simulink model "NewSync_Axial_Flux_Generator_Modelled"  (R2018a)
settings: Solver=ode1  StartTime=0.0  StopTime=1  FixedStep=1e-6  MaxStep=1e-6  RelTol=1e-3
PreLoadFcn:
  | Ts=1/1000
InitFcn:
  | Pref=2000;
  | D=4;
  | P=10;
  | Rd=5;
  | Rq=5;
  | Ld=2.094;
  | Lq= 0.8187;
  | Phi= 1.6
  | Pref = 2000;
  | J=4;
  | K=0.16;
  | c1= 0.5176;
  | c2= 116;
  | c3= 0.4;
  | c4= 5;
  | c5= 21;
  | c6= 0.0068;
  | Den= 1.225;
  | A= 2
  | Ts=1/1000
undefined symbols (not defined in the file): D1, Delta
libraries: powerlib x84, powerlib_meascontrol x17, simulink x13, re_lib x1, electricdrivelib x1, pePowerMeasurement x1
(part 2 of 2)

== system NewSync_Axial_Flux_Generator_Modelled/Utility Grid ==
  120 kV / 25 kV 47 MVA : powerlib/Elements/Three-Phase Transformer (Two Windings)  Winding1Connection=Yg  Winding2Connection=Delta (D1)  CoreType=Three single-phase transformers  SetSaturation=off  Hysteresis=off  DataFile='basic_model'  SetInitialFlux=off  Measurements=None  UNITS=pu  NominalPower=[47e6 60 ]  Winding1="[ 120e3  0.08/30   0.08 ]"  Winding2="[ 25e3  0.08/30  0.08]"  Rm=500  Lm=500  L0=0.5  Saturation="[ 0,0  ;  0.005,1.2  ;  1.0,1.4 ]"  InitialFluxes=[ 0.8 , -0.8 , 0.7 ]  MoreParameters=off  BreakLoop=off  DataType=off  TransfoNumber=0
  120kV 2500MVA : powerlib/Electrical Sources/Three-Phase Source  InternalConnection=Yg  VoltagePhases=off  Voltage=120e3  PhaseAngle=0  Voltage_phases=[25e3 25e3 25e3]/sqrt(3)  PhaseAngles_phases=[0 -120 +120]  Frequency=60  NonIdealSource=on  SpecifyImpedance=on  Resistance=0.8929  Inductance=16.58e-3  ShortCircuitLevel=2500e6  BaseVoltage=120e3  XRratio=7  BusType=swing  Pref=0  Qref=0  Prefabc=[10e3, 10e3, 10e3]  Qrefabc=[0, 0, 0]  Qmin=-inf  Qmax=inf
  14-km Feeder : powerlib/Elements/Distributed Parameters Line  Phases=3  Frequency=60  Resistance=[0.1153 0.413]  Inductance=[1.05e-3 3.32e-3]  Capacitance=[11.33e-009 5.01e-009]  Length=14  x1=[-5.8e-05 -8.35000296312306e-11 0 0;-5.7e-05 -8.31426687600871e-11 0 0;-5.6e-05 -8.27852960725161e-11 0 0;-5.5e-05 -8.24279116193083e-11 0 0;-5.4e-05 -8.2070515451256e-11 0 0;-5.3e-05 -8.1713107619153e-11 0 0;-5.2e-05 -8.13556881737952e-11 0 0;-5.1e-05 -8.09982571659797e-11 0 0;-5e-05 -8.06408146465055e-11 0 0;-4.9e-05 -8.02833606661731e-11 -3803.81447652567 -24026.5579932896;-4.8e-05 -7.99258952757846e-11 -3794.75640746685 -24027.9902901746;-4.7e-05 -7.9568418526144e-11 -3785.69779908852 -24029.4191721463;-4.6e-05 -7.92109304680566e-11 -3776.63865267811 -24030.8446390016;-4.5e-05 -7.88534311523294e-11 -3767.57896952312 -24032.266690538;-4.4e-05 -7.84959206297711e-11 -3758.51875091113 -24033.6853265533;-4.3e-05 -7.81383989511919e-11 -3749.45799812981 -24035.100546846;-4.2e-05 -7.77808661674036e-11 -3740.39671246689 -24036.5123512148;-4.1e-05 -7.74233223292195e-11 -3731.33489521017 -24037.9207394592;-4e-05 -7.70657674874547e-11 -3722.27254764756 -24039.3257113789;-3.9e-05 -7.67082016929256e-11 -3713.209671067 -24040.7272667744;-3.8e-05 -7.63506249964504e-11 -3704.14626675653 -24042.1254054463;-3.7e-05 -7.59930374488485e-11 -3695.08233600428 -24043.5201271961;-3.6e-05 -7.56354391009413e-11 -3686.01788009841 -24044.9114318254;-3.5e-05 -7.52778300035514e-11 -3676.9529003272 -24046.2993191366;-3.4e-05 -7.4920210207503e-11 -3667.88739797898 -24047.6837889324;-3.3e-05 -7.45625797636219e-11 -3658.82137434217 -24049.064841016;-3.2e-05 -7.42049387227354e-11 -3649.75483070523 -24050.4424751912;-3.1e-05 -7.38472871356721e-11 -3640.68776835674 -24051.8166912621;-3e-05 -7.34896250532625e-11 -3631.62018858533 -24053.1874890334;-2.9e-05 -7.31319525263381e-11 -3622.55209267969 -24054.5548683104;-2.8e-05 -7.27742696057324e-11 -3613.48348192861 -24055.9188288987;-2.7e-05 -7.241657634228e-11 -3604.41435762095 -24057.2793706045;-2.6e-05 -7.2058872786817e-11 -3595.34472104562 -24058.6364932343;-2.5e-05 -7.17011589901812e-11 -3586.27457349162 -24059.9901965953;-2.4e-05 -7.13434350032116e-11 -3577.20391624802 -24061.3404804952;-2.3e-05 -7.09857008767488e-11 -3568.13275060397 -24062.6873447419;-2.2e-05 -7.06279566616349e-11 -3559.06107784868 -24064.0307891442;-2.1e-05 -7.02702024087132e-11 -3549.98889927144 -24065.370813511;-2e-05 -6.99124381688286e-11 -3540.91621616161 -24066.7074176519;-1.9e-05 -6.95546639928273e-11 -3531.84302980861 -24068.0406013769;-1.8e-05 -6.91968799315571e-11 -3522.76934150195 -24069.3703644966;-1.7e-05 -6.8839086035867e-11 -3513.69515253121 -24070.6967068221;-1.6e-05 -6.84812823566077e-11 -3504.62046418602 -24072.0196281647;-1.5e-05 -6.81234689446308e-11 -3495.5452777561 -24073.3391283364;-1.4e-05 -6.77656458507897e-11 -3486.46959453125 -24074.6552071498;-1.3e-05 -6.74078131259391e-11 -3477.39341580131 -24075.9678644178;-1.2e-05 -6.70499708209349e-11 -3468.31674285622 -24077.2770999538;-1.1e-05 -6.66921189866345e-11 -3459.23957698596 -24078.5829135718;-1e-05 -6.63342576738967e-11 -3450.16191948062 -24079.8853050861;-9e-06 -6.59763869335815e-11 -3441.08377163032 -24081.1842743117;-8e-06 -6.56185068165503e-11 -3432.00513472528 -24082.479821064;-7e-06 -6.52606173736659e-11 -3422.92601005577 -24083.7719451588;-6e-06 -6.49027186557924e-11 -3413.84639891213 -24085.0606464126;-5e-06 -6.4544810713795e-11 -3404.76630258479 -24086.345924642;-4e-06 -6.41868935985407e-11 -3395.68572236422 -24087.6277796646;-3e-06 -6.38289673608972e-11 -3386.60465954098 -24088.906211298;-2e-06 -6.3471032051734e-11 -3377.5231154057 -24090.1812193606;-1e-06 -6.31130877219217e-11 -3368.44109124905 -24091.4528036713]  x2=[-5.8e-05 -3.28293887343002e-10 0 0;-5.7e-05 -3.27276455725141e-10 0 0;-5.6e-05 -3.26258977593998e-10 0 0;-5.5e-05 -3.25241453094177e-10 0 0;-5.4e-05 -3.24223882370293e-10 0 0;-5.3e-05 -3.23206265566964e-10 0 0;-5.2e-05 -3.22188602828817e-10 0 0;-5.1e-05 -3.21170894300484e-10 0 0;-5e-05 -3.20153140126605e-10 0 0;-4.9e-05 -3.19135340451824e-10 -3384.04949800626 -24234.37909601;-4.8e-05 -3.18117495420794e-10 -3374.91311206833 -24235.653130462;-4.7e-05 -3.17099605178173e-10 -3365.77624647999 -24236.9237204872;-4.6e-05 -3.16081669868627e-10 -3356.63890253978 -24238.190865905;-4.5e-05 -3.15063689636826e-10 -3347.50108154632 -24239.4545665353;-4.4e-05 -3.14045664627449e-10 -3338.36278479831 -24240.7148221985;-4.3e-05 -3.13027594985179e-10 -3329.22401359449 -24241.9716327156;-4.2e-05 -3.12009480854706e-10 -3320.08476923369 -24243.2249979079;-4.1e-05 -3.10991322380728e-10 -3310.9450530148 -24244.4749175972;-4e-05 -3.09973119707947e-10 -3301.80486623678 -24245.7213916059;-3.9e-05 -3.08954872981073e-10 -3292.66421019866 -24246.9644197569;-3.8e-05 -3.07936582344822e-10 -3283.52308619951 -24248.2040018736;-3.7e-05 -3.06918247943915e-10 -3274.38149553851 -24249.4401377796;-3.6e-05 -3.05899869923079e-10 -3265.23943951487 -24250.6728272994;-3.5e-05 -3.0488144842705e-10 -3256.09691942789 -24251.9020702578;-3.4e-05 -3.03862983600568e-10 -3246.95393657692 -24253.12786648;-3.3e-05 -3.0284447558838e-10 -3237.81049226139 -24254.3502157919;-3.2e-05 -3.01825924535237e-10 -3228.66658778077 -24255.5691180197;-3.1e-05 -3.00807330585899e-10 -3219.52222443463 -24256.7845729902;-3e-05 -2.99788693885132e-10 -3210.37740352258 -24257.9965805306;-2.9e-05 -2.98770014577705e-10 -3201.2321263443 -24259.2051404687;-2.8e-05 -2.97751292808395e-10 -3192.08639419954 -24260.4102526328;-2.7e-05 -2.96732528721987e-10 -3182.94020838812 -24261.6119168515;-2.6e-05 -2.95713722463269e-10 -3173.79357020991 -24262.810132954;-2.5e-05 -2.94694874177036e-10 -3164.64648096485 -24264.0049007702;-2.4e-05 -2.93675984008089e-10 -3155.49894195295 -24265.1962201301;-2.3e-05 -2.92657052101235e-10 -3146.35095447428 -24266.3840908645;-2.2e-05 -2.91638078601287e-10 -3137.20251982897 -24267.5685128045;-2.1e-05 -2.90619063653065e-10 -3128.05363931721 -24268.7494857818;-2e-05 -2.89600007401392e-10 -3118.90431423928 -24269.9270096286;-1.9e-05 -2.885809099911e-10 -3109.75454589548 -24271.1010841776;-1.8e-05 -2.87561771567024e-10 -3100.60433558621 -24272.2717092617;-1.7e-05 -2.86542592274007e-10 -3091.45368461191 -24273.4388847147;-1.6e-05 -2.85523372256898e-10 -3082.3025942731 -24274.6026103708;-1.5e-05 -2.8450411166055e-10 -3073.15106587035 -24275.7628860644;-1.4e-05 -2.83484810629823e-10 -3063.9991007043 -24276.9197116308;-1.3e-05 -2.82465469309582e-10 -3054.84670007565 -24278.0730869054;-1.2e-05 -2.81446087844698e-10 -3045.69386528515 -24279.2230117244;-1.1e-05 -2.80426666380049e-10 -3036.54059763362 -24280.3694859243;-1e-05 -2.79407205060516e-10 -3027.38689842196 -24281.5125093423;-9e-06 -2.78387704030988e-10 -3018.2327689511 -24282.6520818158;-8e-06 -2.77368163436359e-10 -3009.07821052206 -24283.7882031829;-7e-06 -2.76348583421528e-10 -2999.9232244359 -24284.9208732821;-6e-06 -2.753289641314e-10 -2990.76781199374 -24286.0500919525;-5e-06 -2.74309305710887e-10 -2981.61197449677 -24287.1758590335;-4e-06 -2.73289608304903e-10 -2972.45571324625 -24288.2981743652;-3e-06 -2.72269872058371e-10 -2963.29902954348 -24289.4170377881;-2e-06 -2.71250097116218e-10 -2954.14192468984 -24290.5324491431;-1e-06 -2.70230283623378e-10 -2944.98439998674 -24291.6444082717]  x3=[-5.8e-05 -9.39139589328699e-11 0 0;-5.7e-05 -9.39069853666868e-11 0 0;-5.6e-05 -9.38999984542268e-11 0 0;-5.5e-05 -9.38929981964829e-11 0 0;-5.4e-05 -9.38859845944499e-11 0 0;-5.3e-05 -9.38789576491248e-11 0 0;-5.2e-05 -9.38719173615061e-11 0 0;-5.1e-05 -9.38648637325944e-11 0 0;-5e-05 -9.38577967633923e-11 0 0;-4.9e-05 -9.3850716454904e-11 -27.3571063473752 -158.181189142487;-4.8e-05 -9.38436228081359e-11 -27.2974715013507 -158.191491287824;-4.7e-05 -9.38365158240962e-11 -27.2378327757468 -158.201770950623;-4.6e-05 -9.38293955037948e-11 -27.1781901790394 -158.212028129421;-4.5e-05 -9.38222618482438e-11 -27.118543719705 -158.222262822762;-4.4e-05 -9.3815114858457e-11 -27.0588934062207 -158.232475029191;-4.3e-05 -9.38079545354501e-11 -26.9992392470643 -158.242664747256;-4.2e-05 -9.38007808802408e-11 -26.9395812507138 -158.25283197551;-4.1e-05 -9.37935938938486e-11 -26.8799194256481 -158.262976712507;-4e-05 -9.3786393577295e-11 -26.8202537803463 -158.273098956805;-3.9e-05 -9.37791799316032e-11 -26.7605843232883 -158.283198706966;-3.8e-05 -9.37719529577985e-11 -26.7009110629545 -158.293275961555;-3.7e-05 -9.37647126569081e-11 -26.6412340078257 -158.303330719139;-3.6e-05 -9.37574590299609e-11 -26.5815531663834 -158.313362978289;-3.5e-05 -9.37501920779878e-11 -26.5218685471097 -158.32337273758;-3.4e-05 -9.37429118020216e-11 -26.4621801584869 -158.333359995588;-3.3e-05 -9.3735618203097e-11 -26.4024880089982 -158.343324750895;-3.2e-05 -9.37283112822506e-11 -26.3427921071271 -158.353267002085;-3.1e-05 -9.37209910405209e-11 -26.2830924613577 -158.363186747743;-3e-05 -9.37136574789482e-11 -26.2233890801748 -158.373083986461;-2.9e-05 -9.37063105985748e-11 -26.1636819720634 -158.382958716832;-2.8e-05 -9.36989504004449e-11 -26.1039711455094 -158.392810937451;-2.7e-05 -9.36915768856045e-11 -26.0442566089988 -158.402640646921;-2.6e-05 -9.36841900551015e-11 -25.9845383710186 -158.412447843842;-2.5e-05 -9.36767899099858e-11 -25.924816440056 -158.422232526821;-2.4e-05 -9.36693764513091e-11 -25.8650908245988 -158.431994694469;-2.3e-05 -9.3661949680125e-11 -25.8053615331354 -158.441734345396;-2.2e-05 -9.36545095974891e-11 -25.7456285741546 -158.451451478219;-2.1e-05 -9.36470562044587e-11 -25.6858919561457 -158.461146091558;-2e-05 -9.36395895020931e-11 -25.6261516875989 -158.470818184034;-1.9e-05 -9.36321094914535e-11 -25.5664077770043 -158.480467754272;-1.8e-05 -9.3624616173603e-11 -25.506660232853 -158.490094800901;-1.7e-05 -9.36171095496065e-11 -25.4469090636365 -158.499699322554;-1.6e-05 -9.3609589620531e-11 -25.3871542778467 -158.509281317864;-1.5e-05 -9.36020563874451e-11 -25.327395883976 -158.51884078547;-1.4e-05 -9.35945098514196e-11 -25.2676338905176 -158.528377724014;-1.3e-05 -9.35869500135268e-11 -25.2078683059649 -158.53789213214;-1.2e-05 -9.35793768748414e-11 -25.1480991388119 -158.547384008496;-1.1e-05 -9.35717904364395e-11 -25.0883263975532 -158.556853351732;-1e-05 -9.35641906993993e-11 -25.0285500906838 -158.566300160504;-9e-06 -9.3556577664801e-11 -24.9687702266993 -158.575724433468;-8e-06 -9.35489513337266e-11 -24.9089868140956 -158.585126169285;-7e-06 -9.35413117072599e-11 -24.8491998613694 -158.594505366619;-6e-06 -9.35336587864867e-11 -24.7894093770178 -158.603862024137;-5e-06 -9.35259925724945e-11 -24.7296153695382 -158.613196140509;-4e-06 -9.35183130663731e-11 -24.6698178474288 -158.622507714408;-3e-06 -9.35106202692138e-11 -24.610016819188 -158.631796744512;-2e-06 -9.35029141821098e-11 -24.5502122933151 -158.641063229499;-1e-06 -9.34951948061565e-11 -24.4904042783094 -158.650307168054]  x4=[-5.8e-05 9.34837785942775e-11 0 0;-5.7e-05 9.34787222842783e-11 0 0;-5.6e-05 9.3473652688868e-11 0 0;-5.5e-05 9.3468569808767e-11 0 0;-5.4e-05 9.34634736446977e-11 0 0;-5.3e-05 9.34583641973845e-11 0 0;-5.2e-05 9.34532414675533e-11 0 0;-5.1e-05 9.34481054559325e-11 0 0;-5e-05 9.34429561632517e-11 0 0;-4.9e-05 9.3437793590243e-11 2.40030560621621 0.492942734397716;-4.8e-05 9.343261773764e-11 2.40011960061937 0.493847593242267;-4.7e-05 9.34274286061783e-11 2.39993325391201 0.494752381900062;-4.6e-05 9.34222261965954e-11 2.39974656612061 0.49565710024251;-4.5e-05 9.34170105096307e-11 2.3995595372717 0.49656174814103;-4.4e-05 9.34117815460254e-11 2.39937216739187 0.497466325467051;-4.3e-05 9.34065393065228e-11 2.39918445650774 0.498370832092013;-4.2e-05 9.34012837918677e-11 2.398996404646 0.499275267887366;-4.1e-05 9.33960150028073e-11 2.39880801183337 0.500179632724568;-4e-05 9.33907329400902e-11 2.39861927809662 0.501083926475089;-3.9e-05 9.33854376044672e-11 2.39843020346258 0.50198814901041;-3.8e-05 9.33801289966909e-11 2.39824078795812 0.502892300202019;-3.7e-05 9.33748071175157e-11 2.39805103161015 0.503796379921417;-3.6e-05 9.3369471967698e-11 2.39786093444566 0.504700388040114;-3.5e-05 9.3364123547996e-11 2.39767049649165 0.50560432442963;-3.4e-05 9.33587618591699e-11 2.39747971777519 0.506508188961496;-3.3e-05 9.33533869019817e-11 2.39728859832339 0.507411981507252;-3.2e-05 9.33479986771952e-11 2.39709713816342 0.508315701938449;-3.1e-05 9.33425971855763e-11 2.39690533732249 0.509219350126649;-3e-05 9.33371824278927e-11 2.39671319582785 0.510122925943423;-2.9e-05 9.33317544049139e-11 2.39652071370682 0.511026429260352;-2.8e-05 9.33263131174113e-11 2.39632789098675 0.51192985994903;-2.7e-05 9.33208585661583e-11 2.39613472769504 0.512833217881057;-2.6e-05 9.33153907519301e-11 2.39594122385915 0.513736502928046;-2.5e-05 9.33099096755037e-11 2.39574737950658 0.514639714961622;-2.4e-05 9.33044153376582e-11 2.39555319466488 0.515542853853417;-2.3e-05 9.32989077391745e-11 2.39535866936164 0.516445919475074;-2.2e-05 9.32933868808352e-11 2.39516380362452 0.517348911698249;-2.1e-05 9.32878527634251e-11 2.3949685974812 0.518251830394606;-2e-05 9.32823053877306e-11 2.39477305095944 0.51915467543582;-1.9e-05 9.32767447545401e-11 2.39457716408701 0.520057446693576;-1.8e-05 9.3271170864644e-11 2.39438093689177 0.520960144039571;-1.7e-05 9.32655837188344e-11 2.3941843694016 0.521862767345511;-1.6e-05 9.32599833179054e-11 2.39398746164443 0.522765316483114;-1.5e-05 9.3254369662653e-11 2.39379021364826 0.523667791324107;-1.4e-05 9.32487427538748e-11 2.39359262544111 0.524570191740227;-1.3e-05 9.32431025923707e-11 2.39339469705107 0.525472517603225;-1.2e-05 9.32374491789422e-11 2.39319642850626 0.526374768784859;-1.1e-05 9.32317825143929e-11 2.39299781983487 0.527276945156899;-1e-05 9.3226102599528e-11 2.39279887106512 0.528179046591127;-9e-06 9.32204094351549e-11 2.39259958222529 0.529081072959332;-8e-06 9.32147030220826e-11 2.3923999533437 0.529983024133318;-7e-06 9.32089833611221e-11 2.39219998444872 0.530884899984896;-6e-06 9.32032504530864e-11 2.39199967556877 0.531786700385891;-5e-06 9.31975042987902e-11 2.39179902673233 0.532688425208135;-4e-06 9.31917448990502e-11 2.3915980379679 0.533590074323475;-3e-06 9.31859722546849e-11 2.39139670930405 0.534491647603765;-2e-06 9.31801863665148e-11 2.3911950407694 0.535393144920871;-1e-06 9.31743872353621e-11 2.3909930323926 0.536294566146672]  x5=5.70973484498186e-05  V1=[0 0 0 5.043e-10 2.433e+04 2.433e+04;0 0 0 377 377 377;1.571 1.571 1.571 1.753 -0.1567 -1.728]  V2=[0 0 0 1.526e-09 2.447e+04 2.447e+04;0 0 0 377 377 377;1.571 1.571 1.571 1.695 -0.1385 -1.709]  I1=[0 0 0 5.598e-11 160.5 160.5;0 0 0 377 377 377;1.571 1.571 1.571 0.4062 -0.171 -1.742]  I2=[0 0 0 5.39e-11 2.45 2.45;0 0 0 377 377 377;1.571 1.571 1.571 -2.748 1.774 0.2028]  nHarmo=2  Measurements=None
      settings: SourceProductName=Simscape Power Systems
  2-MW Load : powerlib/Elements/Three-Phase Parallel RLC Load  LConnTagsString=A|B|C  Configuration=Y (grounded)  NominalVoltage=25e3  Vabc=[1e3 1e3 1e3]  Vabcp=[1e3 1e3 1e3]  NominalFrequency=60  UnbalancedPower=off  ActivePower=2e6  InductivePower=0  CapacitivePower=0  Pabc=[10e3 9e3 11e3]  QLabc=[100 90 110]  QCabc=[100 90 110]  Pabcp=[10e3 9e3 11e3]  QLabcp=[100 90 110]  QCabcp=[100 90 110]  Measurements=None  LoadType=constant Z
  "3.3ohms " : powerlib/Elements/Series RLC Branch  LConnTagsString=__new0  RConnTagsString=__new0  BranchType=R  Resistance=3.3  Inductance=[]  SetiL0=off  InitialCurrent=0  Capacitance=[]  Setx0=off  InitialVoltage=0  Measurements=None
  30-MW 2-Mvar Load : powerlib/Elements/Three-Phase Parallel RLC Load  LConnTagsString=A|B|C  Configuration=Y (grounded)  NominalVoltage=25e3  Vabc=[1e3 1e3 1e3]  Vabcp=[1e3 1e3 1e3]  NominalFrequency=60  UnbalancedPower=off  ActivePower=30e6  InductivePower=2e6  CapacitivePower=0  Pabc=[10e3 9e3 11e3]  QLabc=[100 90 110]  QCabc=[100 90 110]  Pabcp=[10e3 9e3 11e3]  QLabcp=[100 90 110]  QCabcp=[100 90 110]  Measurements=None  LoadType=constant Z
  5-km Feeder : powerlib/Elements/Distributed Parameters Line  Phases=3  Frequency=60  Resistance=[0.1153 0.413]  Inductance=[1.05e-3 3.32e-3]  Capacitance=[11.33e-009 5.01e-009]  Length=5  x1=[-2.1e-05 3.28194991157219e-11 -3553.97109043443 -24057.7583547442;-2e-05 3.29457753731858e-11 -3544.90127687089 -24059.0964606768;-1.9e-05 3.30720469483202e-11 -3535.83095949782 -24060.4311472751;-1.8e-05 3.31983138231792e-11 -3526.76013960432 -24061.7624143496;-1.7e-05 3.33245759798174e-11 -3517.68881847955 -24063.0902617111;-1.6e-05 3.34508334002902e-11 -3508.61699741275 -24064.4146891707;-1.5e-05 3.35770860666536e-11 -3499.54467769323 -24065.7356965404;-1.4e-05 3.37033339609642e-11 -3490.47186061036 -24067.0532836323;-1.3e-05 3.38295770652794e-11 -3481.3985474536 -24068.3674502592;-1.2e-05 3.39558153616572e-11 -3472.32473951246 -24069.6781962344;-1.1e-05 3.40820488321564e-11 -3463.25043807654 -24070.9855213714;-1e-05 3.42082774588364e-11 -3454.17564443549 -24072.2894254846;-9e-06 3.43345012237573e-11 -3445.10035987905 -24073.5899083886;-8e-06 3.44607201089798e-11 -3436.02458569702 -24074.8869698986;-7e-06 3.45869340965654e-11 -3426.94832317927 -24076.1806098303;-6e-06 3.47131431685764e-11 -3417.87157361573 -24077.4708279998;-5e-06 3.48393473070756e-11 -3408.79433829642 -24078.7576242236;-4e-06 3.49655464941265e-11 -3399.71661851141 -24080.0409983191;-3e-06 3.50917407117935e-11 -3390.63841555085 -24081.3209501036;-2e-06 3.52179299421415e-11 -3381.55973070495 -24082.5974793955;-1e-06 3.53441141672363e-11 -3372.480565264 -24083.8705860131]  x2=[-2.1e-05 -6.93589361523303e-11 -3549.98889927144 -24065.370813511;-2e-05 -6.90012549779486e-11 -3540.91621616161 -24066.7074176519;-1.9e-05 -6.86435639969497e-11 -3531.84302980861 -24068.0406013769;-1.8e-05 -6.82858632601694e-11 -3522.76934150195 -24069.3703644966;-1.7e-05 -6.79281528184452e-11 -3513.69515253121 -24070.6967068221;-1.6e-05 -6.75704327226154e-11 -3504.62046418602 -24072.0196281647;-1.5e-05 -6.72127030235203e-11 -3495.5452777561 -24073.3391283364;-1.4e-05 -6.68549637720011e-11 -3486.46959453125 -24074.6552071498;-1.3e-05 -6.64972150189006e-11 -3477.39341580131 -24075.9678644178;-1.2e-05 -6.61394568150628e-11 -3468.31674285622 -24077.2770999538;-1.1e-05 -6.57816892113332e-11 -3459.23957698596 -24078.5829135718;-1e-05 -6.54239122585585e-11 -3450.16191948062 -24079.8853050861;-9e-06 -6.50661260075868e-11 -3441.08377163032 -24081.1842743117;-8e-06 -6.47083305092676e-11 -3432.00513472528 -24082.479821064;-7e-06 -6.43505258144514e-11 -3422.92601005577 -24083.7719451588;-6e-06 -6.39927119739904e-11 -3413.84639891213 -24085.0606464126;-5e-06 -6.36348890387379e-11 -3404.76630258479 -24086.345924642;-4e-06 -6.32770570595485e-11 -3395.68572236422 -24087.6277796646;-3e-06 -6.29192160872781e-11 -3386.60465954098 -24088.906211298;-2e-06 -6.25613661727839e-11 -3377.5231154057 -24090.1812193606;-1e-06 -6.22035073669243e-11 -3368.44109124905 -24091.4528036713]  x3=[-2.1e-05 -9.25400022426598e-11 -14.9168543088507 -81.7615725312542;-2e-05 -9.25349375081922e-11 -14.8860298628988 -81.7671902426389;-1.9e-05 -9.25298596224463e-11 -14.85520330131 -81.7727963330824;-1.8e-05 -9.25247685861438e-11 -14.8243746284655 -81.7783908017878;-1.7e-05 -9.25196644000082e-11 -14.7935438487469 -81.7839736479601;-1.6e-05 -9.25145470647649e-11 -14.7627109665357 -81.7895448708058;-1.5e-05 -9.25094165811413e-11 -14.731875986214 -81.7951044695331;-1.4e-05 -9.25042729498664e-11 -14.7010389121642 -81.8006524433519;-1.3e-05 -9.24991161716714e-11 -14.670199748769 -81.8061887914738;-1.2e-05 -9.24939462472891e-11 -14.6393585004111 -81.8117135131117;-1.1e-05 -9.24887631774542e-11 -14.608515171474 -81.8172266074807;-1e-05 -9.24835669629034e-11 -14.577669766341 -81.822728073797;-9e-06 -9.24783576043753e-11 -14.5468222893961 -81.828217911279;-8e-06 -9.24731351026101e-11 -14.5159727450233 -81.8336961191462;-7e-06 -9.246789945835e-11 -14.4851211376071 -81.8391626966202;-6e-06 -9.24626506723393e-11 -14.4542674715321 -81.8446176429241;-5e-06 -9.24573887453239e-11 -14.4234117511833 -81.8500609572825;-4e-06 -9.24521136780515e-11 -14.3925539809461 -81.8554926389218;-3e-06 -9.2446825471272e-11 -14.3616941652059 -81.8609126870701;-2e-06 -9.24415241257368e-11 -14.3308323083487 -81.8663211009572;-1e-06 -9.24362096421995e-11 -14.2999684147607 -81.8717178798142]  x4=[-2.1e-05 9.37819668971639e-11 -8.89911424191963 -76.0172916483658;-2e-05 9.37768995944502e-11 -8.87045576641855 -76.0206411334412;-1.9e-05 9.37718189639477e-11 -8.84179603022788 -76.0239798142881;-1.8e-05 9.37667250063784e-11 -8.81313503742081 -76.027307690432;-1.7e-05 9.37616177224664e-11 -8.78447279207071 -76.0306247614;-1.6e-05 9.37564971129375e-11 -8.7558092982511 -76.0339310267205;-1.5e-05 9.37513631785194e-11 -8.72714456003573 -76.0372264859238;-1.4e-05 9.37462159199418e-11 -8.69847858149849 -76.0405111385415;-1.3e-05 9.37410553379361e-11 -8.66981136671345 -76.0437849841066;-1.2e-05 9.3735881433236e-11 -8.64114291975486 -76.0470480221541;-1.1e-05 9.37306942065766e-11 -8.61247324469715 -76.05030025222;-1e-05 9.37254936586952e-11 -8.58380234561493 -76.0535416738422;-9e-06 9.3720279790331e-11 -8.55513022658295 -76.05677228656;-8e-06 9.37150526022248e-11 -8.52645689167618 -76.0599920899143;-7e-06 9.37098120951197e-11 -8.49778234496972 -76.0632010834474;-6e-06 9.37045582697604e-11 -8.46910659053888 -76.0663992667033;-5e-06 9.36992911268936e-11 -8.44042963245912 -76.0695866392275;-4e-06 9.36940106672678e-11 -8.41175147480607 -76.0727632005669;-3e-06 9.36887168916337e-11 -8.38307212165554 -76.0759289502702;-2e-06 9.36834098007434e-11 -8.35439157708351 -76.0790838878873;-1e-06 9.36780893953513e-11 -8.32570984516612 -76.0822280129699]  x5=2.03919101606495e-05  V1=[0 0 0 1.661e-10 2.432e+04 2.432e+04;0 0 0 377 377 377;1.571 1.571 1.571 2.066 -0.1453 -1.716]  V2=[0 0 0 5.053e-10 2.433e+04 2.433e+04;0 0 0 377 377 377;1.571 1.571 1.571 1.767 -0.145 -1.716]  I1=[0 0 0 5.154e-11 83.11 83.11;0 0 0 377 377 377;1.571 1.571 1.571 0.3933 -0.179 -1.75]  I2=[0 0 0 5.56e-11 76.54 76.54;0 0 0 377 377 377;1.571 1.571 1.571 -2.784 -0.1151 -1.686]  nHarmo=2  Measurements=None
      settings: SourceProductName=Simscape Power Systems
  Ground3 : powerlib/Elements/Ground  LConnTagsString=a
  "Grounding Transformer " : powerlib/Elements/Grounding Transformer   UNITS=pu  NominalPower="[100e6   60]"  NominalVoltage=25e3  ZeroSequenceImpedance_pu=[0.025 0.75]  MagnetizationBranch_pu=[500 500]  ZeroSequenceImpedance_SI=[0.052083 589.05]  MagnetizationBranch_SI=[1041.7 3.927e+005]  Measurements=None
      settings: SourceProductName=Simscape Power Systems  SourceProductBaseCode=PS
  A : PMIOPort  Side=Left
  B : PMIOPort  Port=2  Side=Left
  C : PMIOPort  Port=3  Side=Left
  connections:
  30-MW 2-Mvar Load/LConn2 -- 14-km Feeder/RConn2 -- 120 kV / 25 kV 47 MVA/RConn2 -- "Grounding Transformer "/LConn2
  "3.3ohms "/RConn1 -- Ground3/LConn1
  30-MW 2-Mvar Load/LConn3 -- 14-km Feeder/RConn3 -- 120 kV / 25 kV 47 MVA/RConn3 -- "Grounding Transformer "/LConn3
  2-MW Load/LConn1 -- 5-km Feeder/RConn1 -- 14-km Feeder/LConn1
  30-MW 2-Mvar Load/LConn1 -- 14-km Feeder/RConn1 -- 120 kV / 25 kV 47 MVA/RConn1 -- "Grounding Transformer "/LConn1
  2-MW Load/LConn3 -- 5-km Feeder/RConn3 -- 14-km Feeder/LConn3
  A/RConn1 -- 5-km Feeder/LConn1
  2-MW Load/LConn2 -- 5-km Feeder/RConn2 -- 14-km Feeder/LConn2
  120 kV / 25 kV 47 MVA/LConn2 -- 120kV 2500MVA/RConn2
  "Grounding Transformer "/RConn1 -- "3.3ohms "/LConn1
  120 kV / 25 kV 47 MVA/LConn1 -- 120kV 2500MVA/RConn1
  C/RConn1 -- 5-km Feeder/LConn3
  120 kV / 25 kV 47 MVA/LConn3 -- 120kV 2500MVA/RConn3
  B/RConn1 -- 5-km Feeder/LConn2

== system NewSync_Axial_Flux_Generator_Modelled/Vd ==
  id : Inport
  iq : Inport  Port=2
  <We> : Inport  Port=3
  Derivative : Derivative
  Gain : Gain  Gain=Ld
  Gain1 : Gain  Gain=Rd
  Gain2 : Gain  Gain=Lq
  Product : Product
  Subtract : Sum  Inputs=--+
  vd : Outport
  wires:
  Derivative/1 -> Gain/1
  Gain1/1 -> Subtract/1
  iq/1 -> Product/1
  Subtract/1 -> vd/1
  id/1 -> Gain1/1, Derivative/1
  Product/1 -> Subtract/3
  <We>/1 -> Gain2/1
  Gain/1 -> Subtract/2
  Gain2/1 -> Product/2

== system NewSync_Axial_Flux_Generator_Modelled/Vq ==
  id : Inport
  <We> : Inport  Port=2
  iq : Inport  Port=3
  Derivative : Derivative
  Gain : Gain  Gain=Ld
  Gain1 : Gain  Gain=Rq
  Gain2 : Gain  Gain=Lq
  Gain3 : Gain  Gain=Phi
  Product : Product
  Subtract : Sum  Inputs=-+--
  vq : Outport
  wires:
  iq/1 -> Gain1/1, Derivative/1
  Product/1 -> Subtract/1
  Gain/1 -> Product/2
  Subtract/1 -> vq/1
  <We>/1 -> Gain3/1, Gain/1
  id/1 -> Product/1
  Gain3/1 -> Subtract/2
  Gain1/1 -> Subtract/3
  Gain2/1 -> Subtract/4
  Derivative/1 -> Gain2/1

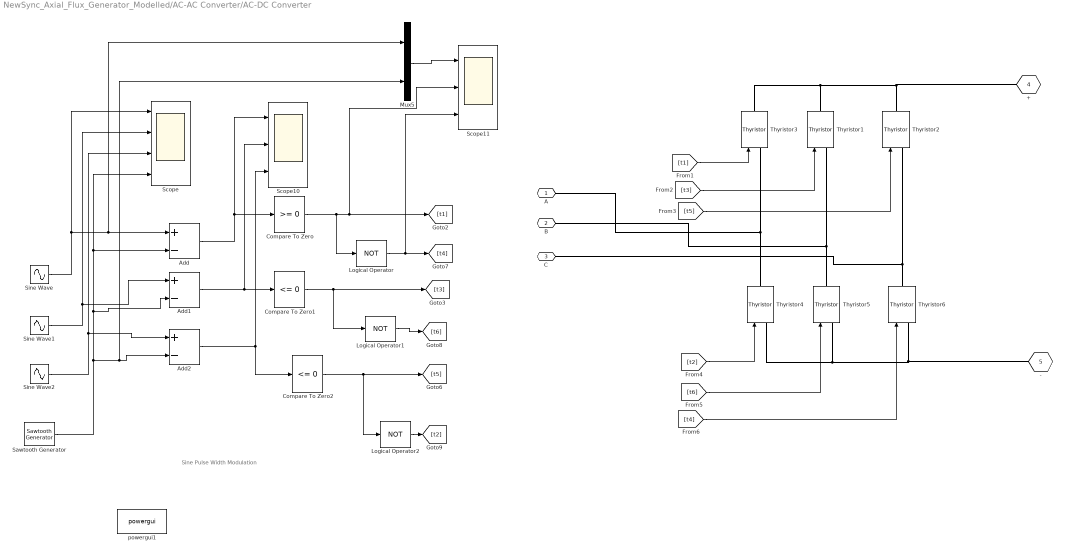
== system NewSync_Axial_Flux_Generator_Modelled/AC-AC Converter/AC-DC Converter ==
  note: Sine Pulse Width Modulation
  Add : Sum  Inputs=+-
  Add1 : Sum  Inputs=+-
  Add2 : Sum  Inputs=+-
  Compare To Zero : simulink/Logic and Bit Operations/Compare To Zero  relop=>=  OutDataTypeStr=boolean
  Compare To Zero1 : simulink/Logic and Bit Operations/Compare To Zero  relop=<=  OutDataTypeStr=boolean
  Compare To Zero2 : simulink/Logic and Bit Operations/Compare To Zero  relop=<=  OutDataTypeStr=boolean
  Logical Operator : Logic  Operator=NOT  AllPortsSameDT=off  OutDataTypeStr=boolean
  Logical Operator1 : Logic  Operator=NOT  AllPortsSameDT=off  OutDataTypeStr=boolean
  Logical Operator2 : Logic  Operator=NOT  AllPortsSameDT=off  OutDataTypeStr=boolean
  Mux5 : Mux  Inputs=2
  Sawtooth Generator : powerlib_meascontrol/Pulse & Signal Generators/Sawtooth Generator  Freq=10  Phase=180  Ts=0
      settings: SourceProductName=Simscape Power Systems
  Scope : Scope  NumInputPorts=4
  Scope10 : Scope  NumInputPorts=3
  Scope11 : Scope  NumInputPorts=3
  Sine Wave : Sin  Frequency=2*pi*60  SampleTime=0
  Sine Wave1 : Sin  Frequency=2*pi*60  Phase=(2*pi)/3  SampleTime=0
  Sine Wave2 : Sin  Frequency=2*pi*60  Phase=(-2*pi)/3  SampleTime=0
  Thyristor{1..6} (6 alike) : powerlib/Power Electronics/Thyristor  Ron=0.001  Lon=0  Vf=0.8  IC=0  Rs=500  Cs=250e-9  Measurements=off
  powergui1 : powerlib/powergui  Priority=1  SimulationMode=Discrete  SampleTime=50e-6  frequency=60  Iterations=50  frequencyindice=0  Pbase=100e6  ErrMax=1e-4  UnitsV=kV  UnitsW=MW  buscounter=0  FunctionMessages=off  echomessages=off  EnableUseOfTLC=off  CurrentSourceSwitches=off  DisableSnubberDevices=off  DisableRonSwitches=off  DisableVfSwitches=off  DisplayEquations=off  SolverType=Tustin/Backward Euler (TBE)  Interpol=off  ExternalGateDelay=off  methode=off  Ts=100  x0status=blocks  SPID=off  SwTol=0  HookPort=off  RestoreLinks=warning  ResistiveCurrentMeasurement=off  Frange=[0:2:500]  Ylog=off  Xlog=on  ShowGrid=off  save=off  variable=ZData  structure=0  ZoomFFT=off  StartTime=0.0  cycles=1  DisplayStyle=1  fundamental=60  FreqAxis=off  MaxFrequency=1000  frequencyindicesteady=1  RmsSteady=1  display=off
  A : PMIOPort  Side=Left
  B : PMIOPort  Port=2  Side=Left
  C : PMIOPort  Port=3  Side=Left
  + : PMIOPort  Port=4  Side=Right
  - : PMIOPort  Port=5  Side=Right
  wires:
  [t5] -> Thyristor2/1
  Logical Operator/1 -> Scope11/3, [t4]
  [t2] -> Thyristor4/1
  Sawtooth Generator/1 -> Mux5/2, Add2/2, Add1/2, Add/2, Scope/4
  Sine Wave1/1 -> Add1/1, Scope/2
  Compare To Zero/1 -> [t1], Scope11/2, Logical Operator/1
  Mux5/1 -> Scope11/1
  [t4] -> Thyristor6/1
  Logical Operator1/1 -> [t6]
  Sine Wave/1 -> Mux5/1, Add/1, Scope/1
  Add2/1 -> Compare To Zero2/1, Scope10/3
  Logical Operator2/1 -> [t2]
  Add1/1 -> Compare To Zero1/1, Scope10/2
  Add/1 -> Scope10/1, Compare To Zero/1
  Compare To Zero1/1 -> Logical Operator1/1, [t3]
  [t1] -> Thyristor3/1
  Sine Wave2/1 -> Add2/1, Scope/3
  Compare To Zero2/1 -> Logical Operator2/1, [t5]
  [t3] -> Thyristor1/1
  [t6] -> Thyristor5/1
  connections:
  Thyristor2/RConn1 -- +/RConn1 -- Thyristor1/RConn1 -- Thyristor3/RConn1
  Thyristor4/LConn1 -- Thyristor5/LConn1 -- -/RConn1 -- Thyristor6/LConn1
  Thyristor3/LConn1 -- A/RConn1 -- Thyristor4/RConn1
  Thyristor6/RConn1 -- C/RConn1 -- Thyristor2/LConn1
  Thyristor5/RConn1 -- B/RConn1 -- Thyristor1/LConn1

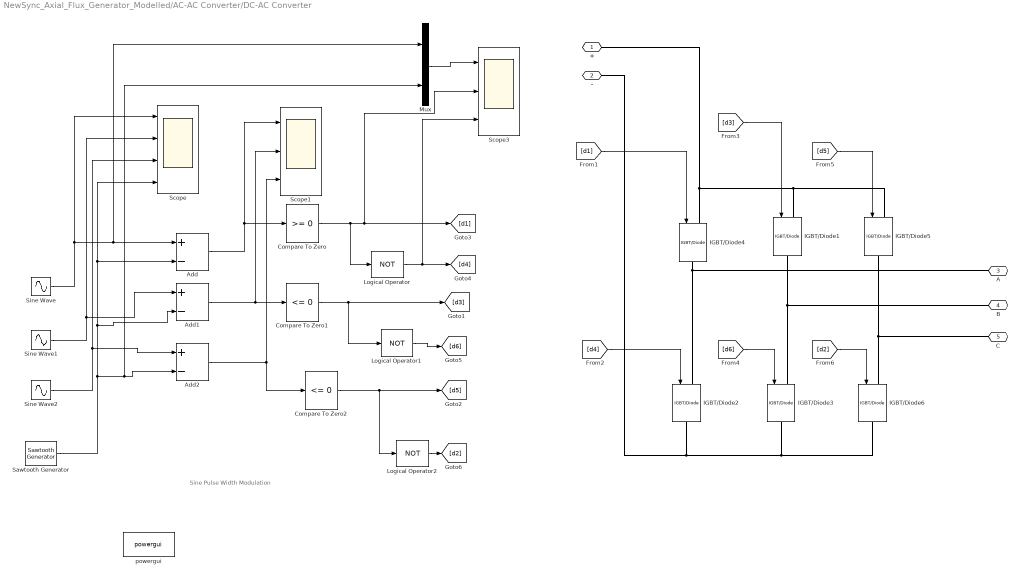
== system NewSync_Axial_Flux_Generator_Modelled/AC-AC Converter/DC-AC Converter ==
  note: Sine Pulse Width Modulation
  Add : Sum  Inputs=+-
  Add1 : Sum  Inputs=+-
  Add2 : Sum  Inputs=+-
  Compare To Zero : simulink/Logic and Bit Operations/Compare To Zero  relop=>=  OutDataTypeStr=boolean
  Compare To Zero1 : simulink/Logic and Bit Operations/Compare To Zero  relop=<=  OutDataTypeStr=boolean
  Compare To Zero2 : simulink/Logic and Bit Operations/Compare To Zero  relop=<=  OutDataTypeStr=boolean
  IGBT/Diode{1..6} (6 alike) : powerlib/Power Electronics/IGBT//Diode  Ron=1e-3  Rs=1e5  Cs=inf  Measurements=off
  Logical Operator : Logic  Operator=NOT  AllPortsSameDT=off  OutDataTypeStr=boolean
  Logical Operator1 : Logic  Operator=NOT  AllPortsSameDT=off  OutDataTypeStr=boolean
  Logical Operator2 : Logic  Operator=NOT  AllPortsSameDT=off  OutDataTypeStr=boolean
  Mux : Mux  Inputs=2
  Sawtooth Generator : powerlib_meascontrol/Pulse & Signal Generators/Sawtooth Generator  Freq=10  Phase=180  Ts=0
      settings: SourceProductName=Simscape Power Systems
  Scope : Scope  NumInputPorts=4
  Scope1 : Scope  NumInputPorts=3
  Scope3 : Scope  NumInputPorts=3
  Sine Wave : Sin  Frequency=2*pi*60  SampleTime=0
  Sine Wave1 : Sin  Frequency=2*pi*60  Phase=(2*pi)/3  SampleTime=0
  Sine Wave2 : Sin  Frequency=2*pi*60  Phase=(-2*pi)/3  SampleTime=0
  powergui : powerlib/powergui  Priority=1  SimulationMode=Discrete  SampleTime=50e-6  frequency=60  Iterations=50  frequencyindice=0  Pbase=100e6  ErrMax=1e-4  UnitsV=kV  UnitsW=MW  buscounter=0  FunctionMessages=off  echomessages=off  EnableUseOfTLC=off  CurrentSourceSwitches=off  DisableSnubberDevices=off  DisableRonSwitches=off  DisableVfSwitches=off  DisplayEquations=off  SolverType=Tustin/Backward Euler (TBE)  Interpol=off  ExternalGateDelay=off  methode=off  Ts=100  x0status=blocks  SPID=off  SwTol=0  HookPort=off  RestoreLinks=warning  ResistiveCurrentMeasurement=off  Frange=[0:2:500]  Ylog=off  Xlog=on  ShowGrid=off  save=off  variable=ZData  structure=0  ZoomFFT=off  StartTime=0.0  cycles=1  DisplayStyle=1  fundamental=60  FreqAxis=off  MaxFrequency=1000  frequencyindicesteady=1  RmsSteady=1  display=off
  + : PMIOPort  Side=Left
  - : PMIOPort  Port=2  Side=Left
  A : PMIOPort  Port=3  Side=Right
  B : PMIOPort  Port=4  Side=Right
  C : PMIOPort  Port=5  Side=Right
  wires:
  Sawtooth Generator/1 -> Mux/2, Add2/2, Add1/2, Add/2, Scope/4
  Add/1 -> Scope1/1, Compare To Zero/1
  Add1/1 -> Compare To Zero1/1, Scope1/2
  Compare To Zero/1 -> [d1], Scope3/2, Logical Operator/1
  [d6] -> IGBT/Diode3/1
  Compare To Zero1/1 -> Logical Operator1/1, [d3]
  Sine Wave/1 -> Mux/1, Add/1, Scope/1
  Sine Wave2/1 -> Add2/1, Scope/3
  Mux/1 -> Scope3/1
  Compare To Zero2/1 -> Logical Operator2/1, [d5]
  [d2] -> IGBT/Diode6/1
  [d1] -> IGBT/Diode4/1
  [d3] -> IGBT/Diode1/1
  [d4] -> IGBT/Diode2/1
  [d5] -> IGBT/Diode5/1
  Add2/1 -> Compare To Zero2/1, Scope1/3
  Sine Wave1/1 -> Add1/1, Scope/2
  Logical Operator2/1 -> [d2]
  Logical Operator1/1 -> [d6]
  Logical Operator/1 -> Scope3/3, [d4]
  connections:
  IGBT/Diode6/LConn1 -- C/RConn1 -- IGBT/Diode5/RConn1
  IGBT/Diode4/RConn1 -- IGBT/Diode2/LConn1 -- A/RConn1
  IGBT/Diode4/LConn1 -- +/RConn1 -- IGBT/Diode5/LConn1 -- IGBT/Diode1/LConn1
  IGBT/Diode6/RConn1 -- -/RConn1 -- IGBT/Diode2/RConn1 -- IGBT/Diode3/RConn1
  IGBT/Diode3/LConn1 -- B/RConn1 -- IGBT/Diode1/RConn1

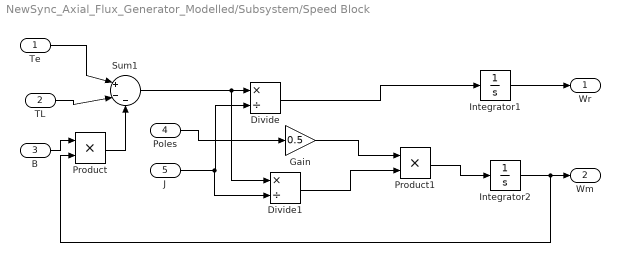
== system NewSync_Axial_Flux_Generator_Modelled/Subsystem/Speed Block ==
  Te : Inport
  TL : Inport  Port=2
  B : Inport  Port=3
  Poles : Inport  Port=4
  J : Inport  Port=5
  Divide : Product  Inputs=*/
  Divide1 : Product  Inputs=*/
  Gain : Gain  Gain=0.5
  Integrator1 : Integrator
  Integrator2 : Integrator
  Product : Product
  Product1 : Product
  Sum1 : Sum  Inputs=|+--
  Wr : Outport
  Wm : Outport  Port=2
  wires:
  Product/1 -> Sum1/3
  Integrator1/1 -> Wr/1
  B/1 -> Product/1
  TL/1 -> Sum1/2
  Integrator2/1 -> Product/2, Wm/1
  Te/1 -> Sum1/1
  Sum1/1 -> Divide1/1, Divide/1
  J/1 -> Divide1/2, Divide/2
  Divide/1 -> Integrator1/1
  Poles/1 -> Gain/1
  Gain/1 -> Product1/1
  Divide1/1 -> Product1/2
  Product1/1 -> Integrator2/1

== system NewSync_Axial_Flux_Generator_Modelled/Subsystem/Te Block ==
  Yq : Inport  Tag=Yq
  Iq : Inport  Port=2
  Yd : Inport  Port=3
  Id : Inport  Port=4
  Poles : Inport  Port=5
  Constant : Constant  Value=3/8
  Fcn : Fcn  Commented=on  Expr=((u(6)*u(5) - u(4)*u(7)) * (3/2)*(u(8)/4))
  Product{,1..2,4} (4 alike) : Product
  Subtract : Sum  Inputs=+-
  Te : Outport
  wires:
  Yd/1 -> Product1/1
  Iq/1 -> Product1/2
  Yq/1 -> Product/1
  Id/1 -> Product/2
  Product1/1 -> Subtract/1
  Product/1 -> Subtract/2
  Subtract/1 -> Product2/1
  Constant/1 -> Product2/2
  Product2/1 -> Product4/1
  Poles/1 -> Product4/2
  Product4/1 -> Te/1

== matlab function NewSync_Axial_Flux_Generator_Modelled/Speed Controller/MATLAB Function ==
  data: w input; y output; t input
function y = fcn(w, t)

A=80;
Tc= 300;

y = A * w * (1-exp(-t/Tc));
